simulink model "ControlBlock_NEWER"  (R2019b)
settings: Solver=FixedStepDiscrete  StartTime=0.0  StopTime=inf  FixedStep=0.01  RelTol=1e-3
values from neighbouring files (symbols this model uses):
  accMax = [15,7.5,10,12.5,15,20,20]'    [initNew.m]
  Kd = 0.1    [MOVE_ABOVE_TABLE.m]    (also in MOVE_ABOVE_TABLE_1.m; initNew.m)
  Kp = 2    [MOVE_ABOVE_TABLE.m]    (also in MOVE_ABOVE_TABLE_1.m; initNew.m = 10)
  pts = single(pts)    [initNew.m]
undefined symbols (not defined in the file or in its folder): DiscIntNeverNeededParam
libraries: simulink_extras x2, xpcutilitieslib x2, xpcrtudplib x2, simulink x1
settings Model: EnablePacing=on  Creator=Aljaz  LastModifiedBy=Aljaz
settings DataIOCC: SaveOutput=off  SaveTime=off  ReturnWorkspaceOutputs=off

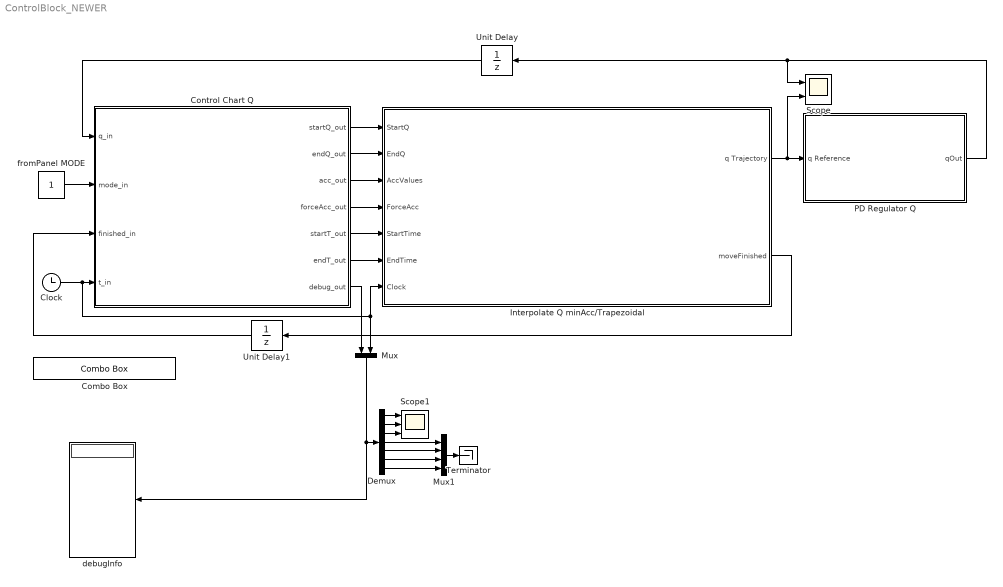
== system ControlBlock_NEWER ==
  Clock : Clock
  Combo Box : ComboBox  LabelPosition=Hide  SelectedLabel=To Default
      settings: Values={{'Hold', 'To Default', 'Planned Motion'}, [0 1 2]}
  Control Chart Q : Stateflow chart  BlockKeywords=__PRM__SERIALIZED__DATA__:Stateflow Chart,Stateflow Diagram  TreatAsAtomicUnit=on
  Demux : Demux  Outputs=7
  Interpolate Q minAcc/Trapezoidal : Subsystem
  Mux : Mux  Inputs=2
  Mux1 : Mux
  PD Regulator Q : Subsystem
  Scope : Scope  NumInputPorts=2
  Scope1 : Scope  NumInputPorts=3
  Terminator : Terminator
  Unit Delay : UnitDelay  InitialCondition=[-pi/6,pi/18,0,-pi/2,0,pi/2,0]'  SampleTime=-1  HasFrameUpgradeWarning=on
  Unit Delay1 : UnitDelay  SampleTime=-1  HasFrameUpgradeWarning=on
  debugInfo : Display
  fromPanel MODE : Constant
  wires:
  Interpolate Q minAcc/Trapezoidal/1(q Trajectory) -> PD Regulator Q/1(q Reference), Scope/2
  Clock/1 -> Interpolate Q minAcc/Trapezoidal/7(Clock), Mux/2, Control Chart Q/4(t_in)
  Control Chart Q/5(startT_out) -> Interpolate Q minAcc/Trapezoidal/5(StartTime)
  Control Chart Q/1(startQ_out) -> Interpolate Q minAcc/Trapezoidal/1(StartQ)
  Control Chart Q/3(acc_out) -> Interpolate Q minAcc/Trapezoidal/3(AccValues)
  Control Chart Q/6(endT_out) -> Interpolate Q minAcc/Trapezoidal/6(EndTime)
  Control Chart Q/2(endQ_out) -> Interpolate Q minAcc/Trapezoidal/2(EndQ)
  PD Regulator Q/1(qOut) -> Unit Delay/1, Scope/1
  fromPanel MODE/1 -> Control Chart Q/2(mode_in)
  Unit Delay/1 -> Control Chart Q/1(q_in)
  Unit Delay1/1 -> Control Chart Q/3(finished_in)
  Interpolate Q minAcc/Trapezoidal/2(moveFinished) -> Unit Delay1/1
  Control Chart Q/7(debug_out) -> Mux/1
  Demux/7 -> Mux1/4
  Demux/4 -> Mux1/1
  Demux/5 -> Mux1/2
  Demux/6 -> Mux1/3
  Mux1/1 -> Terminator/1
  Mux/1 -> Demux/1, debugInfo/1
  Demux/1 -> Scope1/1
  Demux/2 -> Scope1/2
  Demux/3 -> Scope1/3
  Control Chart Q/4(forceAcc_out) -> Interpolate Q minAcc/Trapezoidal/4(ForceAcc)

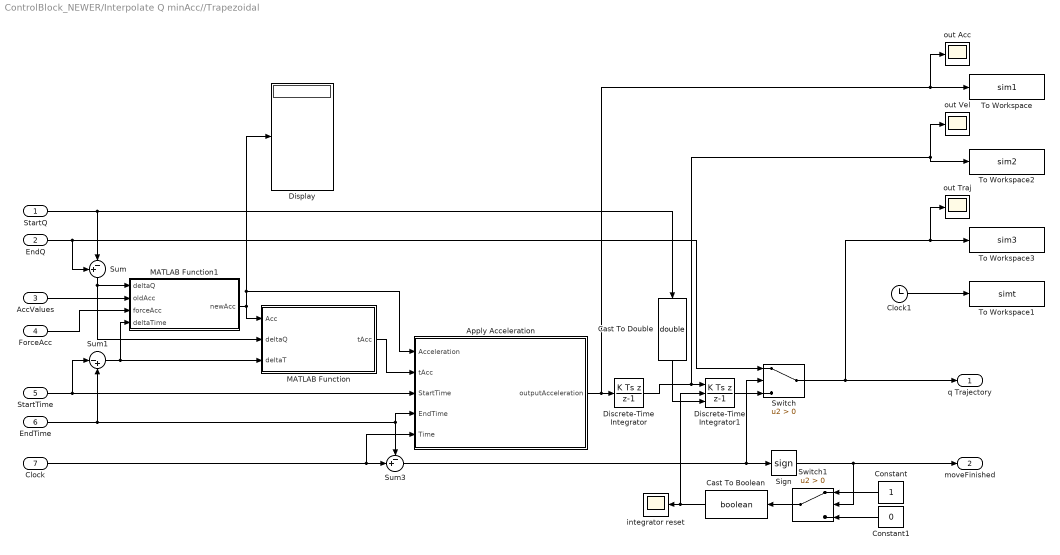
== system ControlBlock_NEWER/Interpolate Q minAcc//Trapezoidal ==
  StartQ : Inport
  EndQ : Inport  Port=2
  AccValues : Inport  Port=3
  ForceAcc : Inport  Port=4
  StartTime : Inport  Port=5
  EndTime : Inport  Port=6
  Clock : Inport  Port=7
  Apply Acceleration : Subsystem
  Cast To Boolean : DataTypeConversion  OutDataTypeStr=boolean
  Cast To Double : DataTypeConversion  OutDataTypeStr=double
  Clock1 : Clock
  Constant : Constant
  Constant1 : Constant  Value=0
  Discrete-Time Integrator : DiscreteIntegrator  IntegratorMethod=Integration: Backward Euler  SampleTime=-1  ICPrevOutput=DiscIntNeverNeededParam  ICPrevScaledInput=DiscIntNeverNeededParam
  Discrete-Time Integrator1 : DiscreteIntegrator  IntegratorMethod=Integration: Backward Euler  ExternalReset=falling  InitialConditionSource=external  SampleTime=-1  ICPrevOutput=DiscIntNeverNeededParam  ICPrevScaledInput=DiscIntNeverNeededParam
  Display : Display
  MATLAB Function : MATLAB Function  TreatAsAtomicUnit=on
  MATLAB Function1 : MATLAB Function  TreatAsAtomicUnit=on
  Sign : Signum
  Sum : Sum  Inputs=+-|
  Sum1 : Sum  Inputs=|-+
  Sum3 : Sum  Inputs=-+|
  Switch : Switch  Criteria=u2 > Threshold
  Switch1 : Switch  Criteria=u2 > Threshold
  To Workspace : ToWorkspace  VariableName=sim1  SampleTime=-1
  To Workspace1 : ToWorkspace  VariableName=simt  SampleTime=-1
  To Workspace2 : ToWorkspace  VariableName=sim2  SampleTime=-1
  To Workspace3 : ToWorkspace  VariableName=sim3  SampleTime=-1
  integrator reset : Scope
  out Acc : Scope
  out Traj : Scope
  out Vel : Scope
  q Trajectory : Outport
  moveFinished : Outport  Port=2
  wires:
  EndTime/1 -> Sum3/1, Apply Acceleration/4(EndTime), Sum1/2
  Sum3/1 -> Switch/2, Sign/1
  ForceAcc/1 -> MATLAB Function1/3(forceAcc)
  MATLAB Function/1(tAcc) -> Apply Acceleration/2(tAcc)
  Clock/1 -> Sum3/2, Apply Acceleration/5(Time)
  Sum1/1 -> MATLAB Function1/4(deltaTime), MATLAB Function/3(deltaT)
  AccValues/1 -> MATLAB Function1/2(oldAcc)
  StartQ/1 -> Cast To Double/1, Sum/2
  StartTime/1 -> Apply Acceleration/3(StartTime), Sum1/1
  Sum/1 -> MATLAB Function1/1(deltaQ), MATLAB Function/2(deltaQ)
  Discrete-Time Integrator1/1 -> Switch/3
  EndQ/1 -> Sum/1, Switch/1
  MATLAB Function1/1(newAcc) -> MATLAB Function/1(Acc), Display/1, Apply Acceleration/1(Acceleration)
  Sign/1 -> Switch1/2, moveFinished/1
  Cast To Boolean/1 -> Discrete-Time Integrator1/2, integrator reset/1
  Cast To Double/1 -> Discrete-Time Integrator1/3
  Switch1/1 -> Cast To Boolean/1
  Constant/1 -> Switch1/1
  Constant1/1 -> Switch1/3
  Apply Acceleration/1(outputAcceleration) -> out Acc/1, To Workspace/1, Discrete-Time Integrator/1
  Clock1/1 -> To Workspace1/1
  Discrete-Time Integrator/1 -> out Vel/1, To Workspace2/1, Discrete-Time Integrator1/1
  Switch/1 -> out Traj/1, To Workspace3/1, q Trajectory/1

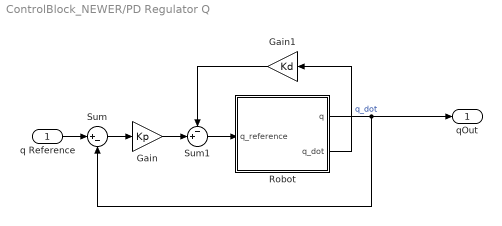
== system ControlBlock_NEWER/PD Regulator Q ==
  q Reference : Inport
  Gain : Gain  Gain=Kp
  Gain1 : Gain  Gain=Kd
  Robot : Subsystem
  Sum : Sum  Inputs=|+-
  Sum1 : Sum  Inputs=-+|
  qOut : Outport
  wires:
  q Reference/1 -> Sum/1
  Sum1/1 -> Robot/1(q_reference)
  Gain/1 -> Sum1/2
  Sum/1 -> Gain/1
  Robot/1(q) -> qOut/1, Sum/2
  Gain1/1 -> Sum1/1
  Robot/2(q_dot) -> Gain1/1  "q_dot"

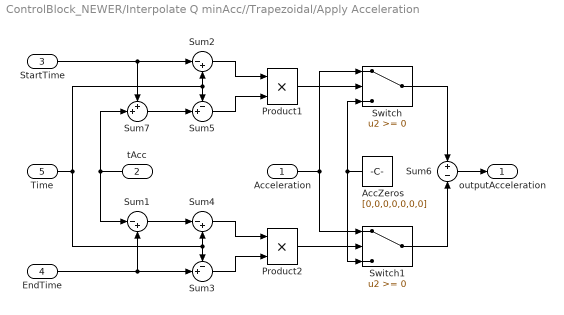
== system ControlBlock_NEWER/Interpolate Q minAcc//Trapezoidal/Apply Acceleration ==
  Acceleration : Inport
  tAcc : Inport  Port=2
  StartTime : Inport  Port=3
  EndTime : Inport  Port=4
  Time : Inport  Port=5
  AccZeros : Constant  Value=[0,0,0,0,0,0,0]
  Product1 : Product
  Product2 : Product
  Sum1 : Sum  Inputs=|-+
  Sum2 : Sum  Inputs=|-+
  Sum3 : Sum  Inputs=-+|
  Sum4 : Sum  Inputs=|-+
  Sum5 : Sum  Inputs=-+|
  Sum6 : Sum  Inputs=+|-
  Sum7 : Sum  Inputs=++|
  Switch : Switch
  Switch1 : Switch
  outputAcceleration : Outport
  wires:
  Switch/1 -> Sum6/1
  Acceleration/1 -> Switch/1, Switch1/1
  Switch1/1 -> Sum6/2
  Product1/1 -> Switch/2
  AccZeros/1 -> Switch/3, Switch1/3
  Sum6/1 -> outputAcceleration/1
  Sum2/1 -> Product1/1
  Sum5/1 -> Product1/2
  Time/1 -> Sum4/2, Sum3/1, Sum2/2, Sum5/1
  StartTime/1 -> Sum7/1, Sum2/1
  tAcc/1 -> Sum1/1, Sum7/2
  Sum7/1 -> Sum5/2
  EndTime/1 -> Sum1/2, Sum3/2
  Sum1/1 -> Sum4/1
  Sum4/1 -> Product2/1
  Sum3/1 -> Product2/2
  Product2/1 -> Switch1/2

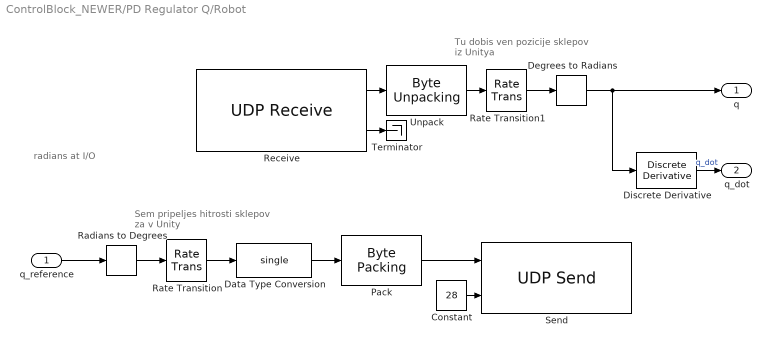
== system ControlBlock_NEWER/PD Regulator Q/Robot ==
  note: radians at I/O
  note: Sem pripeljes hitrosti sklepov za v Unity
  note: Tu dobis ven pozicije sklepov iz Unitya
  q_reference : Inport
  Constant : Constant  Value=28
  Data Type Conversion : DataTypeConversion  OutDataTypeStr=single
  Degrees to Radians : simulink_extras/Transformations/Degrees to Radians
  Discrete Derivative : simulink/Discrete/Discrete Derivative  gainval=1  ICPrevScaledInput=0.0  OutMin=[]  OutMax=[]  OutDataType=fixdt(1, 16)  OutScaling=2^-10  DoSatur=off
  Pack : xpcutilitieslib/Byte Packing   MaskPackedDataType=uint8  MaskUnpackedDataTypes={'single'}  MaskAlignment=1
  Radians to Degrees : simulink_extras/Transformations/Radians to Degrees
  Rate Transition : RateTransition  InitialCondition=[0 0 0 0 0 0 0]
  Rate Transition1 : RateTransition
  Receive : xpcrtudplib/UDP Receive  ipAddressVal=Use host-target connection  localPort=25106  rcvWidth=7*4  rcvFmAny=off  fmAddress=127.0.0.1  rcvMulticast=off  multicastAddress={}  maxUDPQueue=8  sampleTime=0.01
      settings: SourceProductName=Simulink Real-Time
  Send : xpcrtudplib/UDP Send  ipAddressVal=Use host-target connection  localPort=-1  toAddress=127.0.0.1  toPort=25008  sampleTime=0.01
      settings: SourceProductName=Simulink Real-Time  SourceProductBaseCode=XP
  Terminator : Terminator
  Unpack : xpcutilitieslib/Byte Unpacking   MaskUnpackedDataTypes={'single'}  MaskUnpackedDataSizes={[7]}  MaskAlignment=1
      settings: SourceProductName=Simulink Real-Time  SourceProductBaseCode=XP
  q : Outport
  q_dot : Outport  Port=2
  wires:
  Constant/1 -> Send/2
  Pack/1 -> Send/1
  Receive/1 -> Unpack/1
  Rate Transition/1 -> Data Type Conversion/1
  Unpack/1 -> Rate Transition1/1
  Receive/2 -> Terminator/1
  Data Type Conversion/1 -> Pack/1
  Discrete Derivative/1 -> q_dot/1  "q_dot"
  Degrees to Radians/1 -> q/1, Discrete Derivative/1
  Rate Transition1/1 -> Degrees to Radians/1
  q_reference/1 -> Radians to Degrees/1
  Radians to Degrees/1 -> Rate Transition/1

== matlab function ControlBlock_NEWER/Interpolate Q minAcc//Trapezoidal/MATLAB Function1 ==
  data: deltaQ input; oldAcc input; newAcc output; forceAcc input; deltaTime input
function newAcc = adjustAcc(deltaQ,oldAcc,forceAcc,deltaTime)
if forceAcc~=0
    newAcc=oldAcc.*sign(deltaQ); %adjust sign of acc
else
    tAcc=0.49*deltaTime;
    newAcc=(deltaQ./(deltaTime.*tAcc-tAcc.*tAcc));
end
end

== stateflow chart ControlBlock_NEWER/Control Chart Q ==
  state hold
    entry:
    %hold values
    q_hold=q_in;
    t_hold=t_in;
    moveIndex=1;
    finishedState=0;
    %handle outputs
    startQ_out=q_hold;
    endQ_out=q_hold;
    startT_out=t_hold;
    endT_out=t_hold;
    acc_out=accMax;
    forceAcc_out=0;
    debug_out=updateDebug(moveIndex,finishedState,finished_in,startT_out,endT_out,forceAcc_out);
    during:
    %handle outputs
    startQ_out=q_hold;
    endQ_out=q_hold;
    startT_out=t_hold;
    endT_out=t_hold;
    acc_out=accMax;
    forceAcc_out=0;
    debug_out=updateDebug(moveIndex,finishedState,finished_in,startT_out,endT_out,forceAcc_out);
  state toDefault
    entry:
    %hold values
    q_hold=q_in;
    t_hold=t_in;
    moveIndex=1;
    %handle outputs
    startQ_out=q_hold;
    endQ_out=pts(moveIndex,:)';
    startT_out=t_hold;
    endT_out=t_hold+15;
    acc_out=accMax;
    forceAcc_out=0;
    debug_out=updateDebug(moveIndex,finishedState,finished_in,startT_out,endT_out,forceAcc_out);
    during:
    %handle outputs
    startQ_out=q_hold;
    endQ_out=pts(moveIndex,:)';
    startT_out=t_hold;
    endT_out=t_hold+15;
    acc_out=accMax;
    forceAcc_out=0;
    debug_out=updateDebug(moveIndex,finishedState,finished_in,startT_out,endT_out,forceAcc_out);
  state plannedMotion
    entry:
    %hold values
    q_hold=q_in;
    t_hold=t_in;
    moveIndex=1;
    finishedState=0;
    %handle outputs
    startQ_out=q_hold;
    endQ_out=pts(moveIndex,:)';
    startT_out=t_hold;
    endT_out=t_hold+15;
    acc_out=accMax;
    forceAcc_out=0;
    debug_out=updateDebug(moveIndex,finishedState,finished_in,startT_out,endT_out,forceAcc_out);
    during:
    %update move index
    if finished_in==1 && finishedState==0 && moveIndex<size(pts,1)
    moveIndex=moveIndex+1;
    q_hold=q_in;
    t_hold=t_in;
    finishedState=1;
    end
    if finished_in~=1
    finishedState=0;
    end
    %handle outputs
    startQ_out=q_hold;
    endQ_out=pts(moveIndex,:)';
    startT_out=t_hold;
    endT_out=t_hold+15;
    acc_out=accMax;
    forceAcc_out=0;
    debug_out=updateDebug(moveIndex,finishedState,finished_in,startT_out,endT_out,forceAcc_out);
  (default) -> hold
  hold -> toDefault [order 1] : [mode_in==1&&t_in>5]
  toDefault -> hold [order 1] : [mode_in==0]
  hold -> plannedMotion [order 2] : [mode_in==2&&t_in>5]
  plannedMotion -> hold [order 2] : [mode_in==0]
  toDefault -> plannedMotion [order 2] : [mode_in==2]
  plannedMotion -> toDefault [order 1] : [mode_in==1]
  data: moveIdx function_input; internalMoveFinished function_input; externalMoveFinished function_input; tStart function_input; tEnd function_input; forceAcc function_input; debug function_output; q_in input; mode_in input; finished_in input; t_in input; startQ_out output; endQ_out output; acc_out output; forceAcc_out output; startT_out output; endT_out output; q_hold local; pts local single size=[3,7] [1..100]; accMax local size=[7,1]; t_hold local; finishedState local; debug_out output; moveIndex local
  function debug=updateDebug(moveIdx,internalMoveFinished,externalMoveFinished,tStart,tEnd,forceAcc):
    | function  debug=updateDebug(moveIdx,internalMoveFinished,externalMoveFinished,tStart,tEnd,forceAcc)
    | debug=zeros(6,1);
    | debug(1)=moveIdx;
    | debug(2)=internalMoveFinished;
    | debug(3)=externalMoveFinished;
    | debug(4)=tStart;
    | debug(5)=tEnd;
    | debug(6)=forceAcc;

== matlab function ControlBlock_NEWER/Interpolate Q minAcc//Trapezoidal/MATLAB Function ==
  data: Acc input; deltaQ input; tAcc output; deltaT input
function tAcc = getAccTime(Acc,deltaQ,deltaT)

D=deltaT.^2.*Acc-4*deltaQ;
D=D./Acc;
tAcc=deltaT/2-0.5*sqrt(D);
end
